simulink model "Task_01_Sim"  (R2024a)
settings: Solver=VariableStepAuto  StartTime=0.0  StopTime=50.0  RelTol=1e-3
settings Model: Creator=PMYLS  LastModifiedBy=PMYLS

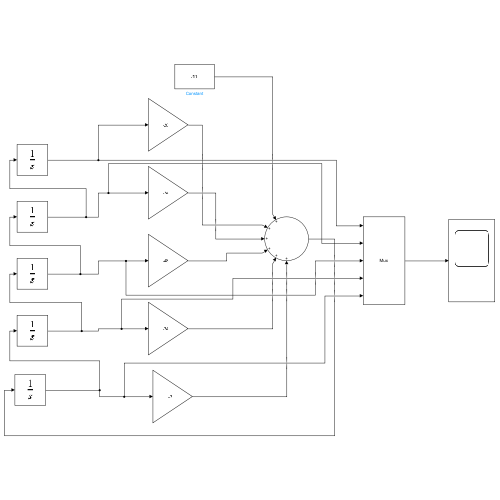
[thumbnail: Simulink's stored preview of the top-level diagram]
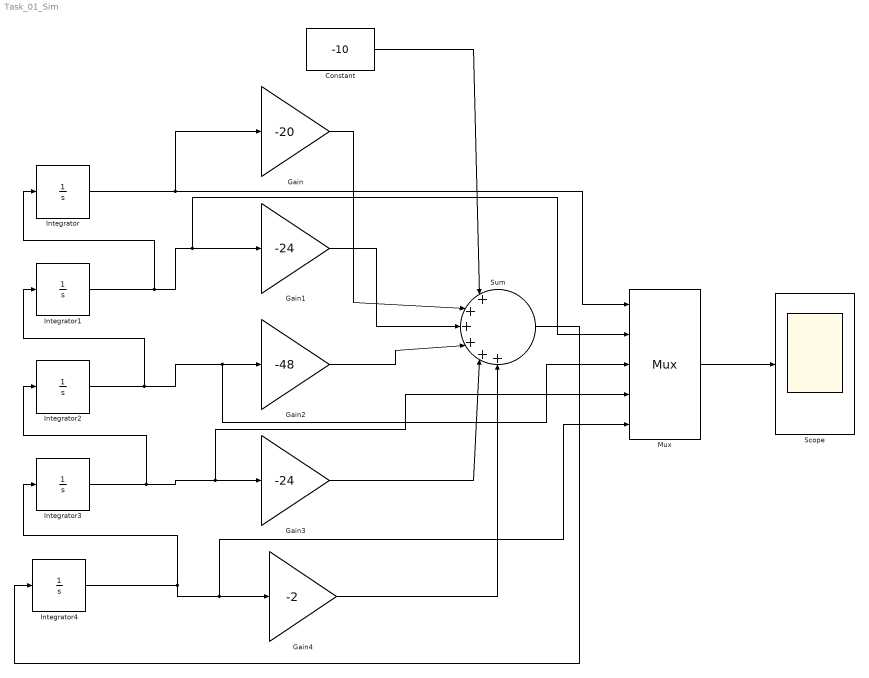
== system Task_01_Sim ==
  Constant : Constant  Value=-10
  Gain : Gain  Gain=-20
  Gain1 : Gain  Gain=-24
  Gain2 : Gain  Gain=-48
  Gain3 : Gain  Gain=-24
  Gain4 : Gain  Gain=-2
  Integrator : Integrator  InitialCondition=2
  Integrator1 : Integrator  InitialCondition=5
  Integrator2 : Integrator  InitialCondition=10
  Integrator3 : Integrator  InitialCondition=-4
  Integrator4 : Integrator  InitialCondition=-7
  Mux : Mux  Inputs=5
  Scope : Scope
  Sum : Sum  Inputs=|++++++
  wires:
  Mux/1 -> Scope/1
  Constant/1 -> Sum/1
  Gain/1 -> Sum/2
  Gain1/1 -> Sum/3
  Gain2/1 -> Sum/4
  Gain3/1 -> Sum/5
  Gain4/1 -> Sum/6
  Integrator/1 -> Mux/1, Gain/1
  Integrator1/1 -> Integrator/1, Mux/2, Gain1/1
  Integrator2/1 -> Integrator1/1, Mux/3, Gain2/1
  Integrator3/1 -> Integrator2/1, Mux/4, Gain3/1
  Integrator4/1 -> Mux/5, Gain4/1, Integrator3/1
  Sum/1 -> Integrator4/1
